simulink library "WECSim_Lib_Body_Elements"  (R2022b)
settings: Solver=VariableStepAuto  StartTime=0.0  StopTime=10.0  RelTol=1e-3
undefined symbols (not defined in the file): body, simu, waves, X, Y, Z
libraries: nesl_utility x24, sm_lib x21, $bdroot x12, vrlib x2
(part 3 of 4)

== system WECSim_Lib_Body_Elements/Rigid Body/Hydrodynamic Body/Wave Diffraction and Excitation Force Calculation/Ramp function ==
  note: The ramp function R, is a smooth function:
      | R = (sin(3*pi/2 + pi * t/Tr) + 1)/2 from t=0 to t=Tr
  Time : Inport
  Add1 : Sum
  Add2 : Sum
  Constant1 : Constant  Value=1/2
  Constant2 : Constant
  Constant3 : Constant  Value=3*pi/2
  Constant4 : Constant  Value=pi
  Divide : Product  Inputs=*/
  Product1 : Product
  Product2 : Product
  Ramp Time : Constant  Value=simu.rampTime
  Sine Wave Function : Sin  TimeSource=Use external signal  SampleTime=0
  R : Outport
  wires:
  Constant1/1 -> Product1/2
  Sine Wave Function/1 -> Add1/2
  Time/1 -> Product2/1
  Product2/1 -> Add2/1
  Add2/1 -> Sine Wave Function/1
  Constant4/1 -> Divide/1
  Add1/1 -> Product1/1
  Divide/1 -> Product2/2  "frequency"
  Ramp Time/1 -> Divide/2  "t_ramp"
  Constant3/1 -> Add2/2  "phase"
  Constant2/1 -> Add1/1
  Product1/1 -> R/1

== system WECSim_Lib_Body_Elements/Rigid Body/Hydrodynamic Body/Wave Radiation Forces Calculation/SS CI and Constant-Damping-CoeVariant Subsystem ==
  note: If the wave type is 'noWave' or 'regular' use constant coefficients.
      | If another wave type and simu.Calc ~= 1, use convolution integral calculation
      | If another wave type and simu.Calc == 1, use the state space calculation
      | If another wave type and simu.FIR == 1, use the FIR filter calculation
  note: 1) Add Subsystem or Model blocks as valid variant choices.
      | 2) You cannot connect blocks at this level. At simulation, connectivity is automatically
      | determined, based on the active variant and port name matching.
  velocity : Inport
  Constant Coefficients : Subsystem  VariantControl=sv_constantCoeff
  Convolution Integral Calculation : Subsystem  VariantControl=sv_convolution
  FIR Filter Calculation : Subsystem  VariantControl=sv_FIR
  "State-Space Calculation " : Subsystem  VariantControl=sv_stateSpace
  Out1 : Outport

== system WECSim_Lib_Body_Elements/Rigid Body/Hydrodynamic Body/Yaw Kinematic Transforms/No B2B ==
  note: If body.yaw.option == 1, interpolate the BEM coefficients to account for the effective change in the incoming wave direction.
  dispGlobal : Inport
  velGlobal : Inport  Port=2
  accGlobal : Inport  Port=3
  Constant : Constant  Value=body.yaw.option
  Yaw Kinematic Transforms : MATLAB Function  TreatAsAtomicUnit=on
  dispLoc : Outport
  velLoc : Outport  Port=2
  accLoc : Outport  Port=3
  wires:
  dispGlobal/1 -> Yaw Kinematic Transforms/2(dispGlobal)
  velGlobal/1 -> Yaw Kinematic Transforms/3(velGlobal)
  accGlobal/1 -> Yaw Kinematic Transforms/4(accGlobal)
  Constant/1 -> Yaw Kinematic Transforms/1(yaw)
  Yaw Kinematic Transforms/2(velLoc) -> velLoc/1
  Yaw Kinematic Transforms/1(dispLoc) -> dispLoc/1
  Yaw Kinematic Transforms/3(accLoc) -> accLoc/1

== system WECSim_Lib_Body_Elements/Rigid Body/Hydrodynamic Body/Yaw Kinematic Transforms/With B2B ==
  note: If body.yaw.option == 1, interpolate the BEM coefficients to account for the effective change in the incoming wave direction.
  dispGlobal : Inport
  velGlobal : Inport  Port=2
  accGlobal : Inport  Port=3
  Constant : Constant  Value=body.yaw.option
  Yaw Kinematic Transforms : MATLAB Function  TreatAsAtomicUnit=on
  dispLoc : Outport
  velLoc : Outport  Port=2
  accLoc : Outport  Port=3
  wires:
  Constant/1 -> Yaw Kinematic Transforms/1(yaw)
  Yaw Kinematic Transforms/1(dispLoc) -> dispLoc/1
  Yaw Kinematic Transforms/2(velLoc) -> velLoc/1
  Yaw Kinematic Transforms/3(accLoc) -> accLoc/1
  dispGlobal/1 -> Yaw Kinematic Transforms/2(dispGlobal)
  velGlobal/1 -> Yaw Kinematic Transforms/3(velGlobal)
  accGlobal/1 -> Yaw Kinematic Transforms/4(accGlobal)

== system WECSim_Lib_Body_Elements/Flex Body/Hydrostatic Restoring Force Calculation/Hydrostatic Restoring Force Calculation/Linear and Nonlinear Restoring Force Variant Subsystem/Linear Hydrostatic Restoring Force ==
  note: The total hydrostatic restoring force is due to a linear stiffness, the vertical buoyancy force (gravity - buoyancy) and a rotational buoyancy force if the center of gravity is not aligned with the center of buoyancy.
      |
      | F_restoring = F_linearRestoringStiffness + F_NetBuoyancy
      |
      | F_linear restoring = hydrostatic restoring coefficient * displacement
      | F_NetBuoyancy = F_gravity - F_buoyancy + F_rotational_buoyancy
      |
      | F_rotational_buoyancy = (cb-cg) x F_buoyancy
      | F_buoyancy = rho*g*V_0
      | F_gravity = m*g
  In1 : Inport
  Add : Sum
  Body Mass : Constant  Value=body.hydroForce.storage.mass
  Linear Restoring Coefficient Matrix : Constant  Value=body.hydroForce.linearHydroRestCoef
  Net Buoyancy Force : Subsystem
  Product2 : Product  Multiplication=Matrix(*)
  Out1 : Outport
  wires:
  Body Mass/1 -> Net Buoyancy Force/1(Body Mass)  "m"
  Net Buoyancy Force/1(F_NetBuoyancy) -> Add/1  "Net buoyancy force"
  Add/1 -> Out1/1  "F_Restoring"
  Linear Restoring Coefficient Matrix/1 -> Product2/1  "K"
  In1/1 -> Product2/2  "x"
  Product2/1 -> Add/2  "Linear Restoring Force"

== system WECSim_Lib_Body_Elements/Flex Body/Hydrostatic Restoring Force Calculation/Hydrostatic Restoring Force Calculation/Linear and Nonlinear Restoring Force Variant Subsystem/Nonlinear Hydrostatic Restoring Force ==
  In1 : Inport
  In2 : Inport  Port=2
  Body Mass : Constant  Value=body.hydroForce.storage.mass
  Center of Gravity : Constant  Value=body.centerGravity
  Gravity : Constant  Value=simu.gravity
  Rate Transition : RateTransition
  Rate Transition1 : RateTransition
  Restoring Forces : MATLAB Function  TreatAsAtomicUnit=on  SystemSampleTime=simu.nonlinearDt
  STL areas : Constant  Value=body.geometry.area
  STL centers : Constant  Value=body.geometry.center
  STL normal vectors : Constant  Value=body.geometry.norm
  To Workspace1 : ToWorkspace  VariableName=body1_hspressure_out  SaveFormat=Structure With Time  SampleTime=-1
      settings: Decimation=round(simu.dtOut/simu.dt,0)
  Water Density : Constant  Value=simu.rho
  Out1 : Outport
  wires:
  Rate Transition/1 -> Out1/1
  Restoring Forces/1(f) -> Rate Transition/1
  Rate Transition1/1 -> To Workspace1/1
  Restoring Forces/2(p) -> Rate Transition1/1
  Body Mass/1 -> Restoring Forces/9(mass)
  STL areas/1 -> Restoring Forces/5(area)
  In2/1 -> Restoring Forces/2(elv)
  STL centers/1 -> Restoring Forces/3(center)
  STL normal vectors/1 -> Restoring Forces/4(tnorm)
  Water Density/1 -> Restoring Forces/6(rho)
  Gravity/1 -> Restoring Forces/7(g)  "g"
  Center of Gravity/1 -> Restoring Forces/8(cg)
  In1/1 -> Restoring Forces/1(x)

== system WECSim_Lib_Body_Elements/Flex Body/Wave Diffraction and Excitation Force Calculation/Wave Diffraction and Excitation Force Calculation/Linear Wave Excitation Force Variant Subsystem/Irregular Wave Excitation Force ==
  note: Calculates the wave force, F_wave, for the case of Irregular Waves.
      |
      | The total force is the combination of the real excitation force, imaginary excitation force, and real part of the mean drift force (fExt.md)
      |
      | F_wave =   sum(A * cos(w * t) * Re{Fext(i)}
      |                            -  A * sin(w * t) * Im{Fext(i)}
      |                            + A * Re(Fext.md(i))
      |                            )
      |
      | where i = each frequency bin
  Time : Inport
  Displacement : Inport  Port=2
  Displacement Phase Enable1 : Constant  Value=body.largeXYDisplacement.option
  Frequency Spacing Delta Omega : Constant  Value=waves.dOmega  VectorParams1D=off
  Imaginary Part of Wave Excitation : Constant  Value=body.hydroForce.fExt.im  VectorParams1D=off
  MATLAB Function : MATLAB Function  TreatAsAtomicUnit=on
  MATLAB Function2 : MATLAB Function  TreatAsAtomicUnit=on
  Random Phase : Constant  Value=waves.phase  VectorParams1D=off
  Real Part of Wave Excitation : Constant  Value=body.hydroForce.fExt.re  VectorParams1D=off
  Real Part of Wave Excitation1 : Constant  Value=body.hydroForce.fExt.md  VectorParams1D=off
  Selector : Selector  IndexOptions=Index vector (dialog)  Indices=[1 2]  OutputSizes=1
  Sum : Sum  Inputs=|++
  Wave Frequency : Constant  Value=waves.omega  VectorParams1D=off
  Wave Spectrum : Constant  Value=waves.amplitude  VectorParams1D=off
  Wave direction : Constant  Value=waves.direction  VectorParams1D=off
  Wave direction spread : Constant  Value=waves.spread  VectorParams1D=off
  Wave number : Constant  Value=waves.wavenumber  VectorParams1D=off
  Linear Excitation : Outport
  wires:
  MATLAB Function/1(Fext) -> Linear Excitation/1
  Wave Frequency/1 -> MATLAB Function2/3(frequency), MATLAB Function/2(w)
  Imaginary Part of Wave Excitation/1 -> MATLAB Function/4(fExtIM)
  Real Part of Wave Excitation/1 -> MATLAB Function/3(fExtRE)
  Wave Spectrum/1 -> MATLAB Function/1(A)
  Time/1 -> MATLAB Function/7(time)
  Frequency Spacing Delta Omega/1 -> MATLAB Function/6(dw)
  Wave direction spread/1 -> MATLAB Function/9(spread)
  Wave direction/1 -> MATLAB Function2/5(direction), MATLAB Function/8(WaveDir)
  Real Part of Wave Excitation1/1 -> MATLAB Function/10(fExtMD)
  Random Phase/1 -> Sum/1
  Sum/1 -> MATLAB Function/5(phaseRand)
  MATLAB Function2/1(dispPhase) -> Sum/2
  Displacement/1 -> Selector/1
  Displacement Phase Enable1/1 -> MATLAB Function2/2(enable)
  Wave number/1 -> MATLAB Function2/4(wavenumber)
  Selector/1 -> MATLAB Function2/1(disp)

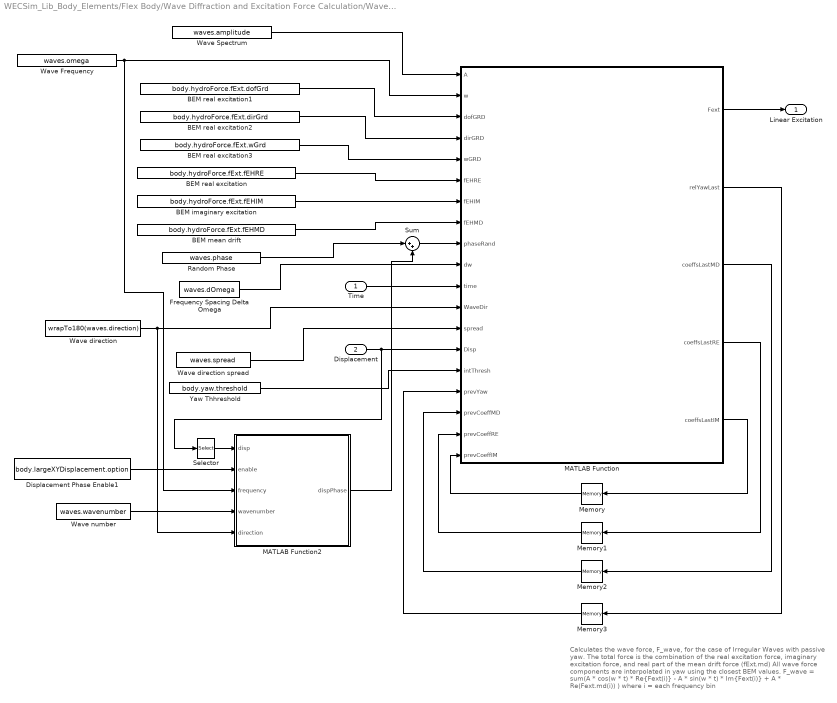
== system WECSim_Lib_Body_Elements/Flex Body/Wave Diffraction and Excitation Force Calculation/Wave Diffraction and Excitation Force Calculation/Linear Wave Excitation Force Variant Subsystem/Irregular Wave NonLinearYaw ==
  note: Calculates the wave force, F_wave, for the case of Irregular Waves with passive yaw.
      |
      | The total force is the combination of the real excitation force, imaginary excitation force, and real part of the mean drift force (fExt.md)
      |
      | All wave force components are interpolated in yaw using the closest BEM values.
      |
      | F_wave =   sum(A * cos(w * t) * Re{Fext(i)}
      |                            -  A * sin(w * t) * Im{Fext(i)}
      |                            + A * Re(Fext.md(i))
      |                            )
      |
      | where i = each frequency bin
  Time : Inport
  Displacement : Inport  Port=2
  BEM imaginary excitation : Constant  Value=body.hydroForce.fExt.fEHIM  VectorParams1D=off
  BEM mean drift : Constant  Value=body.hydroForce.fExt.fEHMD  VectorParams1D=off
  BEM real excitation : Constant  Value=body.hydroForce.fExt.fEHRE  VectorParams1D=off
  BEM real excitation1 : Constant  Value=body.hydroForce.fExt.dofGrd  VectorParams1D=off
  BEM real excitation2 : Constant  Value=body.hydroForce.fExt.dirGrd  VectorParams1D=off
  BEM real excitation3 : Constant  Value=body.hydroForce.fExt.wGrd  VectorParams1D=off
  Displacement Phase Enable1 : Constant  Value=body.largeXYDisplacement.option
  Frequency Spacing Delta Omega : Constant  Value=waves.dOmega  VectorParams1D=off
  MATLAB Function : MATLAB Function  TreatAsAtomicUnit=on
  MATLAB Function2 : MATLAB Function  TreatAsAtomicUnit=on
  Memory{,1..3} (4 alike) : Memory  InheritSampleTime=on  LinearizeAsDelay=on
  Random Phase : Constant  Value=waves.phase  VectorParams1D=off
  Selector : Selector  IndexOptions=Index vector (dialog)  Indices=[1 2]  OutputSizes=1
  Sum : Sum  Inputs=|++
  Wave Frequency : Constant  Value=waves.omega  VectorParams1D=off
  Wave Spectrum : Constant  Value=waves.amplitude  VectorParams1D=off
  Wave direction : Constant  Value=wrapTo180(waves.direction)  VectorParams1D=off
  Wave direction spread : Constant  Value=waves.spread  VectorParams1D=off
  Wave number : Constant  Value=waves.wavenumber  VectorParams1D=off
  Yaw Thhreshold : Constant  Value=body.yaw.threshold
  Linear Excitation : Outport
  wires:
  MATLAB Function/1(Fext) -> Linear Excitation/1
  Memory1/1 -> MATLAB Function/18(prevCoeffRE)
  MATLAB Function/4(coeffsLastRE) -> Memory1/1
  MATLAB Function/2(relYawLast) -> Memory3/1
  Memory2/1 -> MATLAB Function/17(prevCoeffMD)
  BEM real excitation3/1 -> MATLAB Function/5(wGRD)
  BEM real excitation2/1 -> MATLAB Function/4(dirGRD)
  Frequency Spacing Delta Omega/1 -> MATLAB Function/10(dw)
  Wave direction/1 -> MATLAB Function2/5(direction), MATLAB Function/12(WaveDir)
  MATLAB Function/5(coeffsLastIM) -> Memory/1
  Memory3/1 -> MATLAB Function/16(prevYaw)
  BEM imaginary excitation/1 -> MATLAB Function/7(fEHIM)
  Yaw Thhreshold/1 -> MATLAB Function/15(intThresh)
  MATLAB Function/3(coeffsLastMD) -> Memory2/1
  BEM real excitation/1 -> MATLAB Function/6(fEHRE)
  Memory/1 -> MATLAB Function/19(prevCoeffIM)
  Wave Frequency/1 -> MATLAB Function2/3(frequency), MATLAB Function/2(w)
  BEM real excitation1/1 -> MATLAB Function/3(dofGRD)
  Wave Spectrum/1 -> MATLAB Function/1(A)
  BEM mean drift/1 -> MATLAB Function/8(fEHMD)
  Wave direction spread/1 -> MATLAB Function/13(spread)
  Time/1 -> MATLAB Function/11(time)
  Displacement/1 -> Selector/1, MATLAB Function/14(Disp)
  Sum/1 -> MATLAB Function/9(phaseRand)
  Random Phase/1 -> Sum/1
  MATLAB Function2/1(dispPhase) -> Sum/2
  Selector/1 -> MATLAB Function2/1(disp)
  Wave number/1 -> MATLAB Function2/4(wavenumber)
  Displacement Phase Enable1/1 -> MATLAB Function2/2(enable)

== system WECSim_Lib_Body_Elements/Flex Body/Wave Diffraction and Excitation Force Calculation/Wave Diffraction and Excitation Force Calculation/Linear Wave Excitation Force Variant Subsystem/No Wave Excitation Force ==
  Constant : Constant  Value=zeros(1,body.dof)
  Linear Excitation : Outport
  wires:
  Constant/1 -> Linear Excitation/1

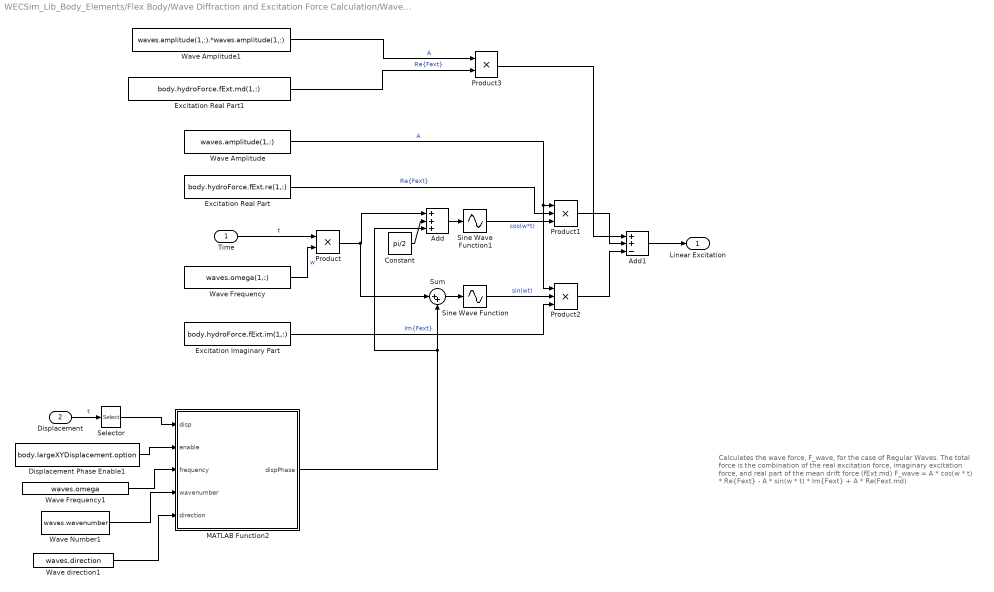
== system WECSim_Lib_Body_Elements/Flex Body/Wave Diffraction and Excitation Force Calculation/Wave Diffraction and Excitation Force Calculation/Linear Wave Excitation Force Variant Subsystem/Regular Wave Excitation Force ==
  note: Calculates the wave force, F_wave, for the case of Regular Waves.
      |
      | The total force is the combination of the real excitation force, imaginary excitation force, and real part of the mean drift force (fExt.md)
      |
      | F_wave =   A * cos(w * t) * Re{Fext}
      |                -  A * sin(w * t) * Im{Fext}
      |                + A * Re(Fext.md)
  Time : Inport
  Displacement : Inport  Port=2
  Add : Sum  Inputs=+++
  Add1 : Sum  Inputs=++-
  Constant : Constant  Value=pi/2
  Displacement Phase Enable1 : Constant  Value=body.largeXYDisplacement.option
  Excitation Imaginary Part : Constant  Value=body.hydroForce.fExt.im(1,:)  VectorParams1D=off
  Excitation Real Part : Constant  Value=body.hydroForce.fExt.re(1,:)  VectorParams1D=off
  Excitation Real Part1 : Constant  Value=body.hydroForce.fExt.md(1,:)  VectorParams1D=off
  MATLAB Function2 : MATLAB Function  TreatAsAtomicUnit=on
  Product : Product
  Product1 : Product  Inputs=3
  Product2 : Product  Inputs=3
  Product3 : Product
  Selector : Selector  IndexOptions=Index vector (dialog)  Indices=[1 2]  OutputSizes=1
  Sine Wave Function : Sin  TimeSource=Use external signal  SampleTime=0
  Sine Wave Function1 : Sin  TimeSource=Use external signal  SampleTime=0
  Sum : Sum  Inputs=|++
  Wave Amplitude : Constant  Value=waves.amplitude(1,:)
  Wave Amplitude1 : Constant  Value=waves.amplitude(1,:).*waves.amplitude(1,:)
  Wave Frequency : Constant  Value=waves.omega(1,:)
  Wave Frequency1 : Constant  Value=waves.omega  VectorParams1D=off
  Wave Number1 : Constant  Value=waves.wavenumber
  Wave direction1 : Constant  Value=waves.direction  VectorParams1D=off
  Linear Excitation : Outport
  wires:
  Time/1 -> Product/1  "t"
  Wave Frequency/1 -> Product/2  "w"
  Product/1 -> Sum/1, Add/1
  Sine Wave Function1/1 -> Product1/3  "cos(w*t)"
  Sine Wave Function/1 -> Product2/2  "sin(wt)"
  Excitation Imaginary Part/1 -> Product2/3  "Im{Fext}"
  Excitation Real Part/1 -> Product1/2  "Re{Fext}"
  Product1/1 -> Add1/2
  Product2/1 -> Add1/3
  Add1/1 -> Linear Excitation/1
  Wave Amplitude/1 -> Product2/1, Product1/1  "A"
  Add/1 -> Sine Wave Function1/1
  Constant/1 -> Add/2
  Wave Amplitude1/1 -> Product3/1  "A"
  Excitation Real Part1/1 -> Product3/2  "Re{Fext}"
  Product3/1 -> Add1/1
  Wave Frequency1/1 -> MATLAB Function2/3(frequency)
  Displacement Phase Enable1/1 -> MATLAB Function2/2(enable)
  Selector/1 -> MATLAB Function2/1(disp)
  Displacement/1 -> Selector/1  "t"
  Wave Number1/1 -> MATLAB Function2/4(wavenumber)
  Wave direction1/1 -> MATLAB Function2/5(direction)
  Sum/1 -> Sine Wave Function/1
  MATLAB Function2/1(dispPhase) -> Add/3, Sum/2

== system WECSim_Lib_Body_Elements/Flex Body/Wave Diffraction and Excitation Force Calculation/Wave Diffraction and Excitation Force Calculation/Linear Wave Excitation Force Variant Subsystem/Regular Wave NonLinear Yaw ==
  note: Calculates the wave force, F_wave, for the case of Regular Waves with passive yaw.
      |
      | The total force is the combination of the real excitation force, imaginary excitation force, and real part of the mean drift force (fExt.md)
      |
      | All wave force components are interpolated in yaw using the closest BEM values.
      |
      | F_wave =   A * cos(w * t) * Re{Fext}
      |                -  A * sin(w * t) * Im{Fext}
      |                + A * Re(Fext.md)
  Time : Inport
  Displacement : Inport  Port=2
  BEM imaginary excitation : Constant  Value=body.hydroForce.fExt.fEHIM  VectorParams1D=off
  BEM imaginary excitation1 : Constant  Value=body.hydroForce.fExt.dirGrd  VectorParams1D=off
  BEM mean drift : Constant  Value=body.hydroForce.fExt.fEHMD  VectorParams1D=off
  BEM real excitation : Constant  Value=body.hydroForce.fExt.fEHRE  VectorParams1D=off
  BEM real excitation1 : Constant  Value=body.hydroForce.fExt.dofGrd  VectorParams1D=off
  Displacement Phase Enable1 : Constant  Value=body.largeXYDisplacement.option
  MATLAB Function2 : MATLAB Function  TreatAsAtomicUnit=on
  MATLAB Function3 : MATLAB Function  TreatAsAtomicUnit=on
  Memory{,1..3} (4 alike) : Memory  InheritSampleTime=on  LinearizeAsDelay=on
  Selector : Selector  IndexOptions=Index vector (dialog)  Indices=[1 2]  OutputSizes=1
  Wave Amplitude : Constant  Value=waves.amplitude(1,:)
  Wave Frequency : Constant  Value=waves.omega(1,:)
  Wave Frequency1 : Constant  Value=waves.omega  VectorParams1D=off
  Wave Number1 : Constant  Value=waves.wavenumber
  Wave direction : Constant  Value=wrapTo180(waves.direction)  VectorParams1D=off
  Wave direction1 : Constant  Value=waves.direction  VectorParams1D=off
  Yaw Threshold : Constant  Value=body.yaw.threshold
  Linear Excitation : Outport
  wires:
  Memory2/1 -> MATLAB Function3/14(prevCoeffMD)
  Yaw Threshold/1 -> MATLAB Function3/11(intThresh)
  BEM imaginary excitation1/1 -> MATLAB Function3/4(dirGRD)
  Memory1/1 -> MATLAB Function3/15(prevCoeffRE)
  BEM real excitation1/1 -> MATLAB Function3/3(dofGRD)
  BEM imaginary excitation/1 -> MATLAB Function3/6(fEHIM)
  Wave direction/1 -> MATLAB Function3/9(WaveDir)
  BEM real excitation/1 -> MATLAB Function3/5(fEHRE)
  MATLAB Function3/3(coeffsLastMD) -> Memory2/1
  Wave Amplitude/1 -> MATLAB Function3/1(A)  "A"
  Memory/1 -> MATLAB Function3/16(prevCoeffIM)
  BEM mean drift/1 -> MATLAB Function3/7(fEHMD)
  Memory3/1 -> MATLAB Function3/13(prevYaw)
  MATLAB Function3/4(coeffsLastRE) -> Memory1/1
  MATLAB Function3/2(relYawLast) -> Memory3/1
  MATLAB Function3/5(coeffsLastIM) -> Memory/1
  Wave Frequency/1 -> MATLAB Function3/2(w)  "w"
  MATLAB Function3/1(Fext) -> Linear Excitation/1
  Time/1 -> MATLAB Function3/8(time)
  Wave Frequency1/1 -> MATLAB Function2/3(frequency)
  Displacement Phase Enable1/1 -> MATLAB Function2/2(enable)
  Selector/1 -> MATLAB Function3/10(Disp), MATLAB Function2/1(disp)
  Displacement/1 -> Selector/1  "t"
  Wave Number1/1 -> MATLAB Function2/4(wavenumber)
  Wave direction1/1 -> MATLAB Function2/5(direction)
  MATLAB Function2/1(dispPhase) -> MATLAB Function3/12(phase)

== system WECSim_Lib_Body_Elements/Flex Body/Wave Diffraction and Excitation Force Calculation/Wave Diffraction and Excitation Force Calculation/Linear Wave Excitation Force Variant Subsystem/User Defined Wave Excitation Force ==
  note: Calculates the wave force, F_wave, for the case of User Defined Waves.
      |
      | F_wave = convolution calculation [1x6]
  InputWaveForceTimeHistory : FromWorkspace  VariableName=[waves.waveAmpTime(:,1),body.hydroForce.userDefinedFe]
  Linear Excitation : Outport
  wires:
  InputWaveForceTimeHistory/1 -> Linear Excitation/1

== system WECSim_Lib_Body_Elements/Flex Body/Wave Diffraction and Excitation Force Calculation/Wave Diffraction and Excitation Force Calculation/Nonlinear FK Force Variant Subsystem/No Nonlinear FroudeKrylov Force ==
  Constant : Constant  Value=zeros(1,body.dof)
  Nonlinear Excitation : Outport
  wires:
  Constant/1 -> Nonlinear Excitation/1

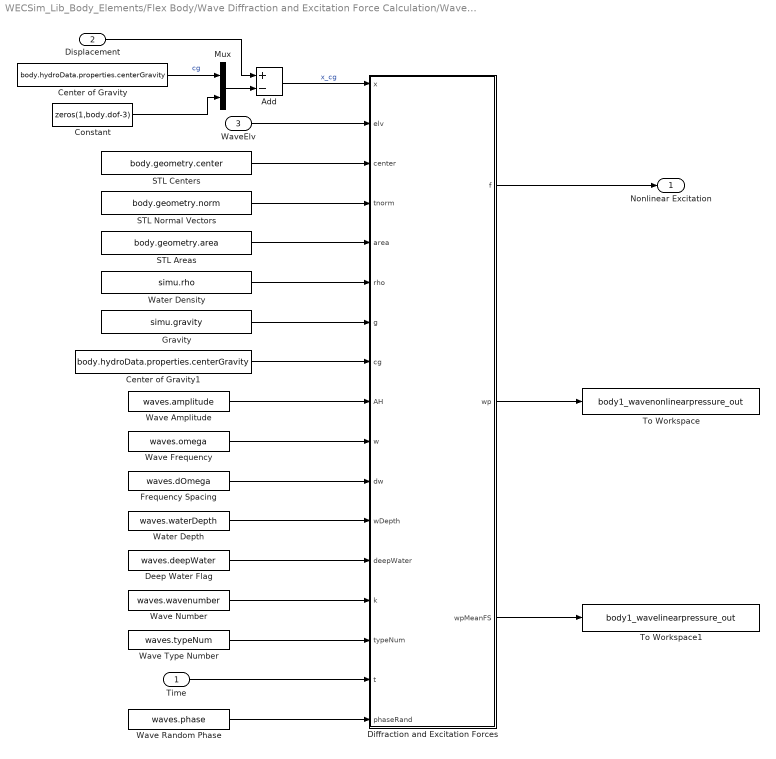
== system WECSim_Lib_Body_Elements/Flex Body/Wave Diffraction and Excitation Force Calculation/Wave Diffraction and Excitation Force Calculation/Nonlinear FK Force Variant Subsystem/With Nonlinear FroudeKrylov Force ==
  Time : Inport
  Displacement : Inport  Port=2
  WaveElv : Inport  Port=3
  Add : Sum  Inputs=+-
  Center of Gravity : Constant  Value=body.hydroData.properties.centerGravity
  Center of Gravity1 : Constant  Value=body.hydroData.properties.centerGravity
  Constant : Constant  Value=zeros(1,body.dof-3)
  Deep Water Flag : Constant  Value=waves.deepWater
  Diffraction and Excitation Forces : MATLAB Function  TreatAsAtomicUnit=on
  Frequency Spacing : Constant  Value=waves.dOmega
  Gravity : Constant  Value=simu.gravity
  Mux : Mux  Inputs=2
  STL Areas : Constant  Value=body.geometry.area
  STL Centers : Constant  Value=body.geometry.center
  STL Normal Vectors : Constant  Value=body.geometry.norm
  To Workspace : ToWorkspace  VariableName=body1_wavenonlinearpressure_out  SaveFormat=Structure With Time  SampleTime=-1
      settings: Decimation=round(simu.dtOut/simu.dt,0)
  To Workspace1 : ToWorkspace  VariableName=body1_wavelinearpressure_out  SaveFormat=Structure With Time  SampleTime=-1
      settings: Decimation=round(simu.dtOut/simu.dt,0)
  Water Density : Constant  Value=simu.rho
  Water Depth : Constant  Value=waves.waterDepth
  Wave Amplitude : Constant  Value=waves.amplitude
  Wave Frequency : Constant  Value=waves.omega
  Wave Number : Constant  Value=waves.wavenumber
  Wave Random Phase : Constant  Value=waves.phase
  Wave Type Number : Constant  Value=waves.typeNum
  Nonlinear Excitation : Outport
  wires:
  Center of Gravity1/1 -> Diffraction and Excitation Forces/8(cg)
  Diffraction and Excitation Forces/1(f) -> Nonlinear Excitation/1
  Gravity/1 -> Diffraction and Excitation Forces/7(g)
  Water Density/1 -> Diffraction and Excitation Forces/6(rho)
  STL Normal Vectors/1 -> Diffraction and Excitation Forces/4(tnorm)
  STL Centers/1 -> Diffraction and Excitation Forces/3(center)
  WaveElv/1 -> Diffraction and Excitation Forces/2(elv)
  Time/1 -> Diffraction and Excitation Forces/16(t)
  Wave Amplitude/1 -> Diffraction and Excitation Forces/9(AH)
  Wave Frequency/1 -> Diffraction and Excitation Forces/10(w)
  Frequency Spacing/1 -> Diffraction and Excitation Forces/11(dw)
  Wave Type Number/1 -> Diffraction and Excitation Forces/15(typeNum)
  Wave Number/1 -> Diffraction and Excitation Forces/14(k)
  Water Depth/1 -> Diffraction and Excitation Forces/12(wDepth)
  Wave Random Phase/1 -> Diffraction and Excitation Forces/17(phaseRand)
  Deep Water Flag/1 -> Diffraction and Excitation Forces/13(deepWater)
  Add/1 -> Diffraction and Excitation Forces/1(x)  "x_cg"
  Mux/1 -> Add/2
  Center of Gravity/1 -> Mux/1  "cg"
  Constant/1 -> Mux/2
  Displacement/1 -> Add/1
  Diffraction and Excitation Forces/3(wpMeanFS) -> To Workspace1/1
  Diffraction and Excitation Forces/2(wp) -> To Workspace/1
  STL Areas/1 -> Diffraction and Excitation Forces/5(area)

== system WECSim_Lib_Body_Elements/Rigid Body/Hydrodynamic Body/B2B Subsystem/B2B/CrossCoupling ==
  note: CrossCoupling block is updated by its mask initialization, which is only called on when a simulation is run. 'From' blocks are automatically created and connected based on the number of bodies in the simulation.
  Mux1 : Mux  Inputs=2
  Mux2 : Mux  Inputs=2
  Transport Delay1 : TransportDelay  DelayTime=10e-8
  Transport Delay2 : TransportDelay  DelayTime=1e-07
  vel : Outport
  acc : Outport  Port=2
  wires:
  [vel1] -> Mux1/1
  Mux1/1 -> vel/1
  [acc1] -> Transport Delay1/1
  Mux2/1 -> acc/1
  Transport Delay1/1 -> Mux2/1
  [vel2] -> Mux1/2
  [acc2] -> Transport Delay2/1
  Transport Delay2/1 -> Mux2/2

== system WECSim_Lib_Body_Elements/Rigid Body/Hydrodynamic Body/Hydrostatic Restoring Force Calculation/Linear and Nonlinear Restoring Force Variant Subsystem/Linear Hydrostatic Restoring Force ==
  note: The total hydrostatic restoring force is due to a linear stiffness, the vertical buoyancy force (gravity - buoyancy) and a rotational buoyancy force if the center of gravity is not aligned with the center of buoyancy.
      |
      | F_restoring = F_linearRestoringStiffness + F_NetBuoyancy
      |
      | F_linear restoring = hydrostatic restoring coefficient * displacement
      | F_NetBuoyancy = F_gravity - F_buoyancy + F_rotational_buoyancy
      |
      | F_rotational_buoyancy = (cb-cg) x F_buoyancy
      | F_buoyancy = rho*g*V_0
      | F_gravity = m*g
  In1 : Inport
  Add : Sum
  Body Mass : Constant  Value=body.hydroForce.storage.mass
  Linear Restoring Coefficient Matrix : Constant  Value=body.hydroForce.linearHydroRestCoef
  Net Buoyancy Force : Subsystem
  Product2 : Product  Multiplication=Matrix(*)
  Out1 : Outport
  wires:
  In1/1 -> Product2/2  "x"
  Linear Restoring Coefficient Matrix/1 -> Product2/1  "K"
  Add/1 -> Out1/1  "F_Restoring"
  Product2/1 -> Add/2  "Linear Restoring Force"
  Net Buoyancy Force/1(F_NetBuoyancy) -> Add/1  "Net buoyancy force"
  Body Mass/1 -> Net Buoyancy Force/1(Body Mass)  "m"

== system WECSim_Lib_Body_Elements/Rigid Body/Hydrodynamic Body/Hydrostatic Restoring Force Calculation/Linear and Nonlinear Restoring Force Variant Subsystem/Nonlinear Hydrostatic Restoring Force ==
  In1 : Inport
  In2 : Inport  Port=2
  Body Mass2 : Constant  Value=body.hydroForce.storage.mass
  Center of Gravity : Constant  Value=body.centerGravity
  Gravity2 : Constant  Value=simu.gravity
  Rate Transition : RateTransition
  Rate Transition1 : RateTransition
  Restoring Forces : MATLAB Function  TreatAsAtomicUnit=on  SystemSampleTime=simu.nonlinearDt
  STL areas : Constant  Value=body.geometry.area
  STL centers : Constant  Value=body.geometry.center
  STL normal vectors : Constant  Value=body.geometry.norm
  To Workspace1 : ToWorkspace  VariableName=body_hspressure_out  SaveFormat=Structure With Time  SampleTime=-1
      settings: Decimation=round(simu.dtOut/simu.dt,0)
  Water Density1 : Constant  Value=simu.rho
  Out1 : Outport
  wires:
  In1/1 -> Restoring Forces/1(x)
  Center of Gravity/1 -> Restoring Forces/8(cg)
  Gravity2/1 -> Restoring Forces/7(g)  "g"
  Water Density1/1 -> Restoring Forces/6(rho)
  STL normal vectors/1 -> Restoring Forces/4(tnorm)
  STL centers/1 -> Restoring Forces/3(center)
  In2/1 -> Restoring Forces/2(elv)
  STL areas/1 -> Restoring Forces/5(area)
  Body Mass2/1 -> Restoring Forces/9(mass)
  Restoring Forces/2(p) -> Rate Transition1/1
  Rate Transition1/1 -> To Workspace1/1
  Restoring Forces/1(f) -> Rate Transition/1
  Rate Transition/1 -> Out1/1

== system WECSim_Lib_Body_Elements/Rigid Body/Hydrodynamic Body/Morison Element and Viscous Damping Force Calculation/Morison Element Variant Subsystem/Morison Element Off ==
  Constant : Constant  Value=zeros(1,body.dof)
  morison_force : Outport
  wires:
  Constant/1 -> morison_force/1

== system WECSim_Lib_Body_Elements/Rigid Body/Hydrodynamic Body/Morison Element and Viscous Damping Force Calculation/Morison Element Variant Subsystem/Morison Element On ==
  note: Chooses the appropriate Morison element variant dependent on the wave type. Note that if passive yaw is used, no block is chosen.
      |
      | If wave.type == 'noWave' | 'noWaveCIC' use No Wave Morison element
      | If wave.type == 'regularWave' | 'regularWaveCIC' use Regular Wave Morison element
      | If wave.type == 'irregularWave' or 'spectrumImport' use Irregular Wave Morison element
  note: 1) Add Subsystem or Model blocks as valid variant choices.
      | 2) You cannot connect blocks at this level. At simulation, connectivity is automatically
      | determined, based on the active variant and port name matching.
  displacement : Inport
  velocity : Inport  Port=2
  acceleration : Inport  Port=3
  time : Inport  Port=4
  Irregular Wave Morison Force : Subsystem  TreatAsAtomicUnit=on  SystemSampleTime=simu.morisonDt  VariantControl=sv_irregularWaves_b1
  No Wave Morison Force : Subsystem  VariantControl=sv_noWave
  Regular Wave Morison Force : Subsystem  TreatAsAtomicUnit=on  SystemSampleTime=simu.morisonDt  VariantControl=sv_regularWaves_b1
  morison_force : Outport

== system WECSim_Lib_Body_Elements/Rigid Body/Hydrodynamic Body/Nonlinear Wave Elevation/Linear or Instantaneous Free Surface/Instantaneous Water Free Surface ==
  note: Calculate the instantaneous wave elevation for the nonlinear hydrodynamics options.
  In1 : Inport
  In2 : Inport  Port=2
  Center of Gravity : Constant  Value=body.centerGravity
  Frequency Spacing : Constant  Value=waves.dOmega
  Instantaneous FS : MATLAB Function  TreatAsAtomicUnit=on
  Ramp Time : Constant  Value=simu.rampTime
  STL Centers : Constant  Value=body.geometry.center
  Wave Amplitude : Constant  Value=waves.amplitude
  Wave Direction : Constant  Value=waves.direction
  Wave Frequency : Constant  Value=waves.omega
  Wave Number : Constant  Value=waves.wavenumber
  Wave Random Phase : Constant  Value=waves.phase
  Wave Type Number : Constant  Value=waves.typeNum
  Out1 : Outport
  wires:
  Instantaneous FS/1(f) -> Out1/1
  STL Centers/1 -> Instantaneous FS/2(center)
  Center of Gravity/1 -> Instantaneous FS/3(cg)
  Wave Number/1 -> Instantaneous FS/7(k)
  Wave Frequency/1 -> Instantaneous FS/5(w)
  Wave Type Number/1 -> Instantaneous FS/8(typeNum)
  Ramp Time/1 -> Instantaneous FS/10(rampT)
  Wave Random Phase/1 -> Instantaneous FS/11(phaseRand)
  Frequency Spacing/1 -> Instantaneous FS/6(dw)
  In2/1 -> Instantaneous FS/9(t)
  In1/1 -> Instantaneous FS/1(x)
  Wave Direction/1 -> Instantaneous FS/12(waveDir)
  Wave Amplitude/1 -> Instantaneous FS/4(AH)

== system WECSim_Lib_Body_Elements/Rigid Body/Hydrodynamic Body/Nonlinear Wave Elevation/Linear or Instantaneous Free Surface/Mean Water Free Surface ==
  note: The mean water surface is always zero.
  zero : Constant  Value=0
  Out1 : Outport
  wires:
  zero/1 -> Out1/1

== system WECSim_Lib_Body_Elements/Rigid Body/Hydrodynamic Body/Wave Diffraction and Excitation Force Calculation/Linear Wave Excitation Force Variant Subsystem/Irregular Wave Excitation Force ==
  note: Calculates the wave force, F_wave, for the case of Irregular Waves.
      |
      | The total force is the combination of the real excitation force, imaginary excitation force, and real part of the mean drift force (fExt.md)
      |
      | F_wave =   sum(A * cos(w * t) * Re{Fext(i)}
      |                            -  A * sin(w * t) * Im{Fext(i)}
      |                            + A * Re(Fext.md(i))
      |                            )
      |
      | where i = each frequency bin
  Time : Inport
  Displacement : Inport  Port=2
  Displacement Phase Enable1 : Constant  Value=body.largeXYDisplacement.option
  Frequency Spacing Delta Omega : Constant  Value=waves.dOmega  VectorParams1D=off
  Imaginary Part of Wave Excitation : Constant  Value=body.hydroForce.fExt.im  VectorParams1D=off
  MATLAB Function : MATLAB Function  TreatAsAtomicUnit=on
  MATLAB Function2 : MATLAB Function  TreatAsAtomicUnit=on
  Random Phase : Constant  Value=waves.phase  VectorParams1D=off
  Real Part of Wave Excitation : Constant  Value=body.hydroForce.fExt.re  VectorParams1D=off
  Real Part of Wave Excitation1 : Constant  Value=body.hydroForce.fExt.md  VectorParams1D=off
  Selector : Selector  IndexOptions=Index vector (dialog)  Indices=[1 2]  OutputSizes=1
  Sum : Sum  Inputs=|++
  Wave Frequency : Constant  Value=waves.omega  VectorParams1D=off
  Wave Frequency1 : Constant  Value=waves.omega  VectorParams1D=off
  Wave Number1 : Constant  Value=waves.wavenumber
  Wave Spectrum : Constant  Value=waves.amplitude  VectorParams1D=off
  Wave direction spread : Constant  Value=waves.spread  VectorParams1D=off
  Wave direction1 : Constant  Value=waves.direction  VectorParams1D=off
  Linear Excitation : Outport
  wires:
  MATLAB Function/1(Fext) -> Linear Excitation/1
  Wave Frequency/1 -> MATLAB Function/2(w)
  Imaginary Part of Wave Excitation/1 -> MATLAB Function/4(fExtIM)
  Real Part of Wave Excitation/1 -> MATLAB Function/3(fExtRE)
  Wave Spectrum/1 -> MATLAB Function/1(A)
  Time/1 -> MATLAB Function/7(time)
  Frequency Spacing Delta Omega/1 -> MATLAB Function/6(dw)
  Wave direction spread/1 -> MATLAB Function/9(spread)
  Real Part of Wave Excitation1/1 -> MATLAB Function/10(fExtMD)
  MATLAB Function2/1(dispPhase) -> Sum/2
  Sum/1 -> MATLAB Function/5(phaseRand)
  Random Phase/1 -> Sum/1
  Wave Frequency1/1 -> MATLAB Function2/3(frequency)
  Displacement Phase Enable1/1 -> MATLAB Function2/2(enable)
  Selector/1 -> MATLAB Function2/1(disp)
  Displacement/1 -> Selector/1  "t"
  Wave Number1/1 -> MATLAB Function2/4(wavenumber)
  Wave direction1/1 -> MATLAB Function/8(WaveDir), MATLAB Function2/5(direction)

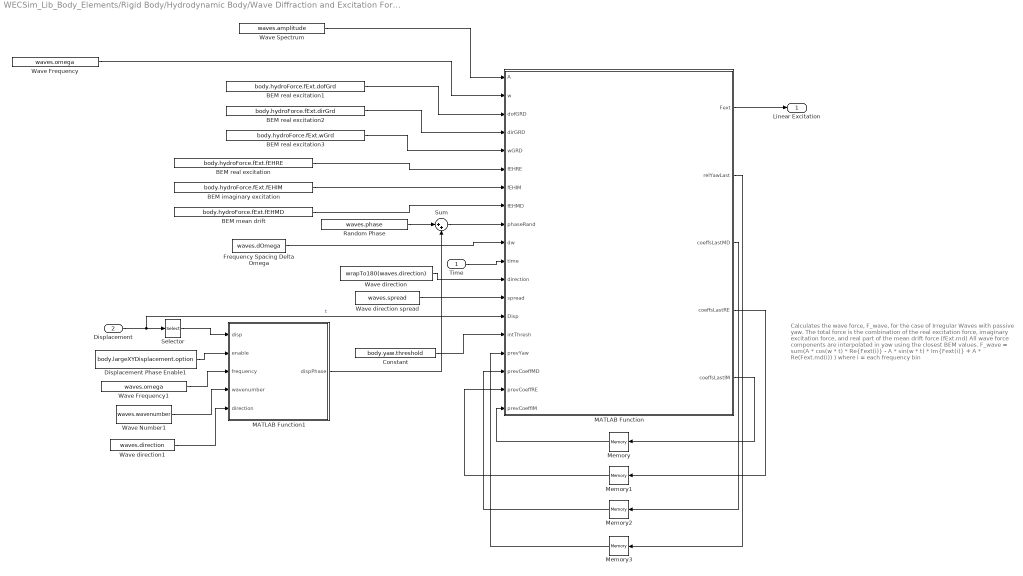
== system WECSim_Lib_Body_Elements/Rigid Body/Hydrodynamic Body/Wave Diffraction and Excitation Force Calculation/Linear Wave Excitation Force Variant Subsystem/Irregular Wave NonLinearYaw ==
  note: Calculates the wave force, F_wave, for the case of Irregular Waves with passive yaw.
      |
      | The total force is the combination of the real excitation force, imaginary excitation force, and real part of the mean drift force (fExt.md)
      |
      | All wave force components are interpolated in yaw using the closest BEM values.
      |
      | F_wave =   sum(A * cos(w * t) * Re{Fext(i)}
      |                            -  A * sin(w * t) * Im{Fext(i)}
      |                            + A * Re(Fext.md(i))
      |                            )
      |
      | where i = each frequency bin
  Time : Inport
  Displacement : Inport  Port=2
  BEM imaginary excitation : Constant  Value=body.hydroForce.fExt.fEHIM  VectorParams1D=off
  BEM mean drift : Constant  Value=body.hydroForce.fExt.fEHMD  VectorParams1D=off
  BEM real excitation : Constant  Value=body.hydroForce.fExt.fEHRE  VectorParams1D=off
  BEM real excitation1 : Constant  Value=body.hydroForce.fExt.dofGrd  VectorParams1D=off
  BEM real excitation2 : Constant  Value=body.hydroForce.fExt.dirGrd  VectorParams1D=off
  BEM real excitation3 : Constant  Value=body.hydroForce.fExt.wGrd  VectorParams1D=off
  Constant : Constant  Value=body.yaw.threshold
  Displacement Phase Enable1 : Constant  Value=body.largeXYDisplacement.option
  Frequency Spacing Delta Omega : Constant  Value=waves.dOmega  VectorParams1D=off
  MATLAB Function : MATLAB Function  TreatAsAtomicUnit=on
  MATLAB Function1 : MATLAB Function  TreatAsAtomicUnit=on
  Memory{,1..3} (4 alike) : Memory  InheritSampleTime=on  LinearizeAsDelay=on
  Random Phase : Constant  Value=waves.phase  VectorParams1D=off
  Selector : Selector  IndexOptions=Index vector (dialog)  Indices=[1 2]  OutputSizes=1
  Sum : Sum  Inputs=|++
  Wave Frequency : Constant  Value=waves.omega  VectorParams1D=off
  Wave Frequency1 : Constant  Value=waves.omega  VectorParams1D=off
  Wave Number1 : Constant  Value=waves.wavenumber
  Wave Spectrum : Constant  Value=waves.amplitude  VectorParams1D=off
  Wave direction : Constant  Value=wrapTo180(waves.direction)  VectorParams1D=off
  Wave direction spread : Constant  Value=waves.spread  VectorParams1D=off
  Wave direction1 : Constant  Value=waves.direction  VectorParams1D=off
  Linear Excitation : Outport
  wires:
  MATLAB Function/1(Fext) -> Linear Excitation/1
  Memory1/1 -> MATLAB Function/18(prevCoeffRE)
  MATLAB Function/4(coeffsLastRE) -> Memory1/1
  MATLAB Function/2(relYawLast) -> Memory3/1
  Memory2/1 -> MATLAB Function/17(prevCoeffMD)
  BEM real excitation3/1 -> MATLAB Function/5(wGRD)
  BEM real excitation2/1 -> MATLAB Function/4(dirGRD)
  Frequency Spacing Delta Omega/1 -> MATLAB Function/10(dw)
  Wave direction/1 -> MATLAB Function/12(direction)
  MATLAB Function/5(coeffsLastIM) -> Memory/1
  Memory3/1 -> MATLAB Function/16(prevYaw)
  BEM imaginary excitation/1 -> MATLAB Function/7(fEHIM)
  Constant/1 -> MATLAB Function/15(intThresh)
  MATLAB Function/3(coeffsLastMD) -> Memory2/1
  BEM real excitation/1 -> MATLAB Function/6(fEHRE)
  Memory/1 -> MATLAB Function/19(prevCoeffIM)
  Wave Frequency/1 -> MATLAB Function/2(w)
  BEM real excitation1/1 -> MATLAB Function/3(dofGRD)
  Wave Spectrum/1 -> MATLAB Function/1(A)
  BEM mean drift/1 -> MATLAB Function/8(fEHMD)
  Wave direction spread/1 -> MATLAB Function/13(spread)
  Time/1 -> MATLAB Function/11(time)
  Random Phase/1 -> Sum/1
  Sum/1 -> MATLAB Function/9(phaseRand)
  Wave Frequency1/1 -> MATLAB Function1/3(frequency)
  Displacement Phase Enable1/1 -> MATLAB Function1/2(enable)
  Selector/1 -> MATLAB Function1/1(disp)
  Displacement/1 -> MATLAB Function/14(Disp), Selector/1  "t"
  Wave Number1/1 -> MATLAB Function1/4(wavenumber)
  Wave direction1/1 -> MATLAB Function1/5(direction)
  MATLAB Function1/1(dispPhase) -> Sum/2

== system WECSim_Lib_Body_Elements/Rigid Body/Hydrodynamic Body/Wave Diffraction and Excitation Force Calculation/Linear Wave Excitation Force Variant Subsystem/No Wave Excitation Force ==
  Constant : Constant  Value=zeros(1,body.dof)
  Linear Excitation : Outport
  wires:
  Constant/1 -> Linear Excitation/1

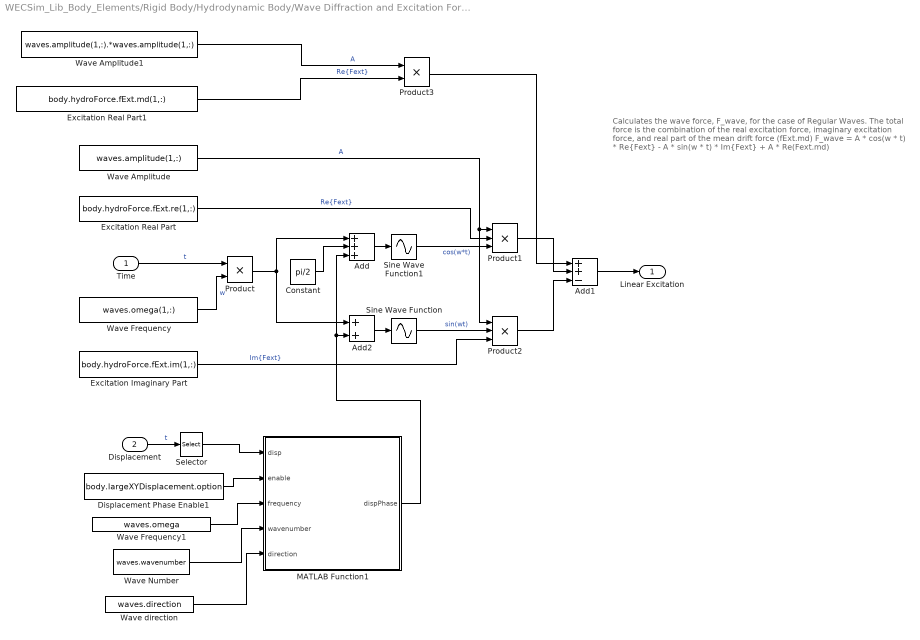
== system WECSim_Lib_Body_Elements/Rigid Body/Hydrodynamic Body/Wave Diffraction and Excitation Force Calculation/Linear Wave Excitation Force Variant Subsystem/Regular Wave Excitation Force ==
  note: Calculates the wave force, F_wave, for the case of Regular Waves.
      |
      | The total force is the combination of the real excitation force, imaginary excitation force, and real part of the mean drift force (fExt.md)
      |
      | F_wave =   A * cos(w * t) * Re{Fext}
      |                -  A * sin(w * t) * Im{Fext}
      |                + A * Re(Fext.md)
  Time : Inport
  Displacement : Inport  Port=2
  Add : Sum  Inputs=+++
  Add1 : Sum  Inputs=++-
  Add2 : Sum
  Constant : Constant  Value=pi/2
  Displacement Phase Enable1 : Constant  Value=body.largeXYDisplacement.option
  Excitation Imaginary Part : Constant  Value=body.hydroForce.fExt.im(1,:)  VectorParams1D=off
  Excitation Real Part : Constant  Value=body.hydroForce.fExt.re(1,:)  VectorParams1D=off
  Excitation Real Part1 : Constant  Value=body.hydroForce.fExt.md(1,:)  VectorParams1D=off
  MATLAB Function1 : MATLAB Function  TreatAsAtomicUnit=on
  Product : Product
  Product1 : Product  Inputs=3
  Product2 : Product  Inputs=3
  Product3 : Product
  Selector : Selector  IndexOptions=Index vector (dialog)  Indices=[1 2]  OutputSizes=1
  Sine Wave Function : Sin  TimeSource=Use external signal  SampleTime=0
  Sine Wave Function1 : Sin  TimeSource=Use external signal  SampleTime=0
  Wave Amplitude : Constant  Value=waves.amplitude(1,:)
  Wave Amplitude1 : Constant  Value=waves.amplitude(1,:).*waves.amplitude(1,:)
  Wave Frequency : Constant  Value=waves.omega(1,:)
  Wave Frequency1 : Constant  Value=waves.omega  VectorParams1D=off
  Wave Number : Constant  Value=waves.wavenumber
  Wave direction : Constant  Value=waves.direction  VectorParams1D=off
  Linear Excitation : Outport
  wires:
  Time/1 -> Product/1  "t"
  Wave Frequency/1 -> Product/2  "w"
  Product/1 -> Add2/1, Add/1
  Sine Wave Function1/1 -> Product1/3  "cos(w*t)"
  Sine Wave Function/1 -> Product2/2  "sin(wt)"
  Excitation Imaginary Part/1 -> Product2/3  "Im{Fext}"
  Excitation Real Part/1 -> Product1/2  "Re{Fext}"
  Product1/1 -> Add1/2
  Product2/1 -> Add1/3
  Add1/1 -> Linear Excitation/1
  Wave Amplitude/1 -> Product2/1, Product1/1  "A"
  Add/1 -> Sine Wave Function1/1
  Constant/1 -> Add/2
  Wave Amplitude1/1 -> Product3/1  "A"
  Excitation Real Part1/1 -> Product3/2  "Re{Fext}"
  Product3/1 -> Add1/1
  Displacement/1 -> Selector/1  "t"
  Displacement Phase Enable1/1 -> MATLAB Function1/2(enable)
  MATLAB Function1/1(dispPhase) -> Add/3, Add2/2
  Add2/1 -> Sine Wave Function/1
  Selector/1 -> MATLAB Function1/1(disp)
  Wave Frequency1/1 -> MATLAB Function1/3(frequency)
  Wave Number/1 -> MATLAB Function1/4(wavenumber)
  Wave direction/1 -> MATLAB Function1/5(direction)

== system WECSim_Lib_Body_Elements/Rigid Body/Hydrodynamic Body/Wave Diffraction and Excitation Force Calculation/Linear Wave Excitation Force Variant Subsystem/Regular Wave NonLinear Yaw ==
  note: Calculates the wave force, F_wave, for the case of Regular Waves with passive yaw.
      |
      | The total force is the combination of the real excitation force, imaginary excitation force, and real part of the mean drift force (fExt.md)
      |
      | All wave force components are interpolated in yaw using the closest BEM values.
      |
      | F_wave =   A * cos(w * t) * Re{Fext}
      |                -  A * sin(w * t) * Im{Fext}
      |                + A * Re(Fext.md)
  Time : Inport
  Displacement : Inport  Port=2
  BEM imaginary excitation : Constant  Value=body.hydroForce.fExt.fEHIM  VectorParams1D=off
  BEM imaginary excitation1 : Constant  Value=body.hydroForce.fExt.dirGrd  VectorParams1D=off
  BEM mean drift : Constant  Value=body.hydroForce.fExt.fEHMD  VectorParams1D=off
  BEM real excitation : Constant  Value=body.hydroForce.fExt.fEHRE  VectorParams1D=off
  BEM real excitation1 : Constant  Value=body.hydroForce.fExt.dofGrd  VectorParams1D=off
  Constant : Constant  Value=body.yaw.threshold
  Displacement Phase Enable1 : Constant  Value=body.largeXYDisplacement.option
  MATLAB Function1 : MATLAB Function  TreatAsAtomicUnit=on
  MATLAB Function3 : MATLAB Function  TreatAsAtomicUnit=on
  Memory{,1..3} (4 alike) : Memory  InheritSampleTime=on  LinearizeAsDelay=on
  Selector : Selector  IndexOptions=Index vector (dialog)  Indices=[1 2]  OutputSizes=1
  Wave Amplitude : Constant  Value=waves.amplitude(1,:)
  Wave Frequency : Constant  Value=waves.omega(1,:)
  Wave Frequency1 : Constant  Value=waves.omega  VectorParams1D=off
  Wave Number1 : Constant  Value=waves.wavenumber
  Wave direction : Constant  Value=wrapTo180(waves.direction)  VectorParams1D=off
  Wave direction1 : Constant  Value=waves.direction  VectorParams1D=off
  Linear Excitation : Outport
  wires:
  Memory2/1 -> MATLAB Function1/14(prevCoeffMD)
  Constant/1 -> MATLAB Function1/11(intThresh)
  BEM imaginary excitation1/1 -> MATLAB Function1/4(dirGRD)
  Memory1/1 -> MATLAB Function1/15(prevCoeffRE)
  BEM real excitation1/1 -> MATLAB Function1/3(dofGRD)
  BEM imaginary excitation/1 -> MATLAB Function1/6(fEHIM)
  Wave direction/1 -> MATLAB Function1/9(WaveDir)
  BEM real excitation/1 -> MATLAB Function1/5(fEHRE)
  MATLAB Function1/3(coeffsLastMD) -> Memory2/1
  Wave Amplitude/1 -> MATLAB Function1/1(A)  "A"
  Memory/1 -> MATLAB Function1/16(prevCoeffIM)
  BEM mean drift/1 -> MATLAB Function1/7(fEHMD)
  Memory3/1 -> MATLAB Function1/13(prevYaw)
  MATLAB Function1/4(coeffsLastRE) -> Memory1/1
  MATLAB Function1/2(relYawLast) -> Memory3/1
  MATLAB Function1/5(coeffsLastIM) -> Memory/1
  Wave Frequency/1 -> MATLAB Function1/2(w)  "w"
  MATLAB Function1/1(Fext) -> Linear Excitation/1
  Time/1 -> MATLAB Function1/8(time)
  MATLAB Function3/1(dispPhase) -> MATLAB Function1/12(phase)
  Wave direction1/1 -> MATLAB Function3/5(direction)
  Displacement/1 -> MATLAB Function1/10(Disp), Selector/1  "t"
  Wave Number1/1 -> MATLAB Function3/4(wavenumber)
  Displacement Phase Enable1/1 -> MATLAB Function3/2(enable)
  Selector/1 -> MATLAB Function3/1(disp)
  Wave Frequency1/1 -> MATLAB Function3/3(frequency)

== system WECSim_Lib_Body_Elements/Rigid Body/Hydrodynamic Body/Wave Diffraction and Excitation Force Calculation/Linear Wave Excitation Force Variant Subsystem/User Defined Wave Excitation Force ==
  note: Calculates the wave force, F_wave, for the case of User Defined Waves.
      |
      | F_wave = convolution calculation [1x6]
  InputWaveForceTimeHistory : FromWorkspace  VariableName=[waves.waveAmpTime(:,1),body.hydroForce.userDefinedFe]
  Linear Excitation : Outport
  wires:
  InputWaveForceTimeHistory/1 -> Linear Excitation/1

== system WECSim_Lib_Body_Elements/Rigid Body/Hydrodynamic Body/Wave Diffraction and Excitation Force Calculation/Nonlinear FK Force Variant Subsystem/No Nonlinear FroudeKrylov Force ==
  Constant : Constant  Value=zeros(1,body.dof)
  Nonlinear Excitation : Outport
  wires:
  Constant/1 -> Nonlinear Excitation/1

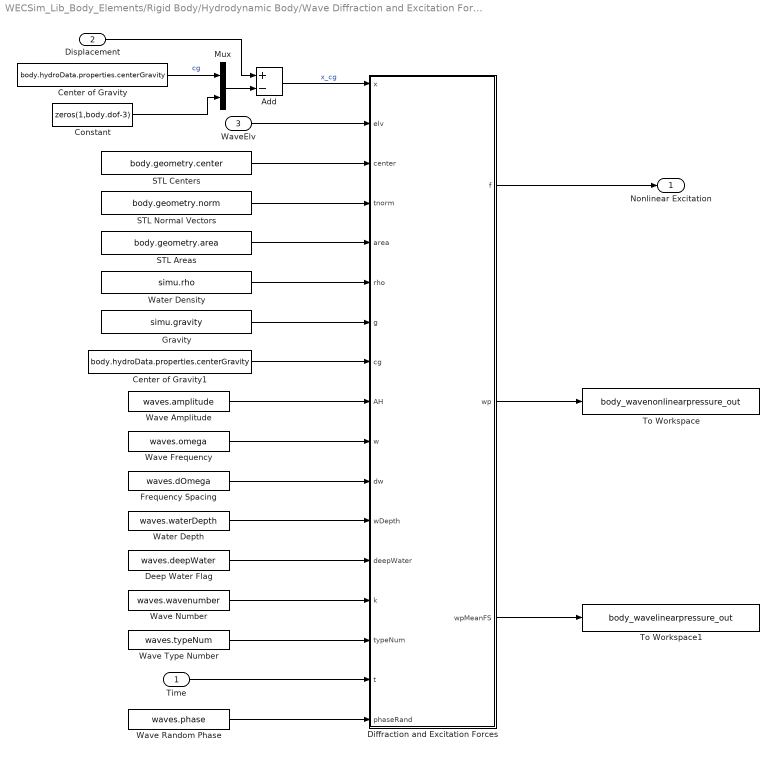
== system WECSim_Lib_Body_Elements/Rigid Body/Hydrodynamic Body/Wave Diffraction and Excitation Force Calculation/Nonlinear FK Force Variant Subsystem/With Nonlinear FroudeKrylov Force ==
  Time : Inport
  Displacement : Inport  Port=2
  WaveElv : Inport  Port=3
  Add : Sum  Inputs=+-
  Center of Gravity : Constant  Value=body.hydroData.properties.centerGravity
  Center of Gravity1 : Constant  Value=body.hydroData.properties.centerGravity
  Constant : Constant  Value=zeros(1,body.dof-3)
  Deep Water Flag : Constant  Value=waves.deepWater
  Diffraction and Excitation Forces : MATLAB Function  TreatAsAtomicUnit=on
  Frequency Spacing : Constant  Value=waves.dOmega
  Gravity : Constant  Value=simu.gravity
  Mux : Mux  Inputs=2
  STL Areas : Constant  Value=body.geometry.area
  STL Centers : Constant  Value=body.geometry.center
  STL Normal Vectors : Constant  Value=body.geometry.norm
  To Workspace : ToWorkspace  VariableName=body_wavenonlinearpressure_out  SaveFormat=Structure With Time  SampleTime=-1
      settings: Decimation=round(simu.dtOut/simu.dt,0)
  To Workspace1 : ToWorkspace  VariableName=body_wavelinearpressure_out  SaveFormat=Structure With Time  SampleTime=-1
      settings: Decimation=round(simu.dtOut/simu.dt,0)
  Water Density : Constant  Value=simu.rho
  Water Depth : Constant  Value=waves.waterDepth
  Wave Amplitude : Constant  Value=waves.amplitude
  Wave Frequency : Constant  Value=waves.omega
  Wave Number : Constant  Value=waves.wavenumber
  Wave Random Phase : Constant  Value=waves.phase
  Wave Type Number : Constant  Value=waves.typeNum
  Nonlinear Excitation : Outport
  wires:
  Center of Gravity1/1 -> Diffraction and Excitation Forces/8(cg)
  Diffraction and Excitation Forces/1(f) -> Nonlinear Excitation/1
  Gravity/1 -> Diffraction and Excitation Forces/7(g)
  Water Density/1 -> Diffraction and Excitation Forces/6(rho)
  STL Normal Vectors/1 -> Diffraction and Excitation Forces/4(tnorm)
  STL Centers/1 -> Diffraction and Excitation Forces/3(center)
  WaveElv/1 -> Diffraction and Excitation Forces/2(elv)
  Time/1 -> Diffraction and Excitation Forces/16(t)
  Wave Amplitude/1 -> Diffraction and Excitation Forces/9(AH)
  Wave Frequency/1 -> Diffraction and Excitation Forces/10(w)
  Frequency Spacing/1 -> Diffraction and Excitation Forces/11(dw)
  Wave Type Number/1 -> Diffraction and Excitation Forces/15(typeNum)
  Wave Number/1 -> Diffraction and Excitation Forces/14(k)
  Water Depth/1 -> Diffraction and Excitation Forces/12(wDepth)
  Wave Random Phase/1 -> Diffraction and Excitation Forces/17(phaseRand)
  Deep Water Flag/1 -> Diffraction and Excitation Forces/13(deepWater)
  Add/1 -> Diffraction and Excitation Forces/1(x)  "x_cg"
  Mux/1 -> Add/2
  Center of Gravity/1 -> Mux/1  "cg"
  Constant/1 -> Mux/2
  Displacement/1 -> Add/1
  Diffraction and Excitation Forces/3(wpMeanFS) -> To Workspace1/1
  Diffraction and Excitation Forces/2(wp) -> To Workspace/1
  STL Areas/1 -> Diffraction and Excitation Forces/5(area)

== system WECSim_Lib_Body_Elements/Rigid Body/Hydrodynamic Body/Wave Radiation Forces Calculation/SS CI and Constant-Damping-CoeVariant Subsystem/Constant Coefficients ==
  note: F = damping * velocity
  velocity : Inport
  Product : Product  Multiplication=Matrix(*)
  Radiation Damping Matrix : Constant  Value=body.hydroForce.fDamping
  Out1 : Outport
  wires:
  Radiation Damping Matrix/1 -> Product/1
  Product/1 -> Out1/1  "F_Single Frequency"
  velocity/1 -> Product/2

== system WECSim_Lib_Body_Elements/Rigid Body/Hydrodynamic Body/Wave Radiation Forces Calculation/SS CI and Constant-Damping-CoeVariant Subsystem/Convolution Integral Calculation ==
  note: Calculate the convolution integral using the radiation IRF (body.hydroForce.irkb) and the velocity.
  velocity : Inport
  IRBK : Constant  Value=body.hydroForce.irkb
  MATLAB Function1 : MATLAB Function  TreatAsAtomicUnit=on  SystemSampleTime=simu.cicTime(2)-simu.cicTime(1)
  Rate Transition : RateTransition
  Reshape : Reshape
  cicTime : Constant  Value=simu.cicTime
  Out1 : Outport
  wires:
  Reshape/1 -> Out1/1
  Rate Transition/1 -> Reshape/1
  MATLAB Function1/1(F_FM) -> Rate Transition/1
  IRBK/1 -> MATLAB Function1/2(IRKB)
  cicTime/1 -> MATLAB Function1/3(cicTime)
  velocity/1 -> MATLAB Function1/1(velocity)
